simulink model "task1"  (R2024a)
settings: Solver=FixedStepAuto  StartTime=0.0  StopTime=10  FixedStep=0.001  RelTol=1e-3
settings Model: Creator=eva  LastModifiedBy=eva

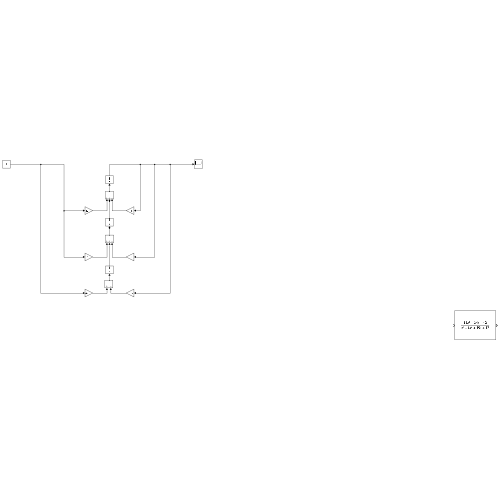
[thumbnail: Simulink's stored preview of the top-level diagram]
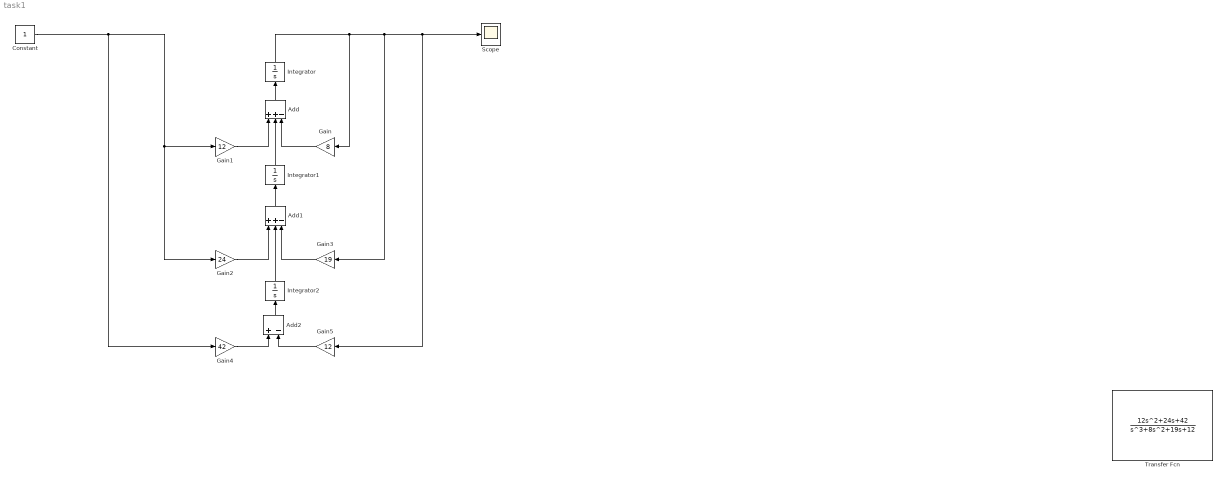
== system task1 ==
  Add : Sum  Inputs=++-
  Add1 : Sum  Inputs=++-
  Add2 : Sum  Inputs=+-
  Constant : Constant
  Gain : Gain  Gain=8
  Gain1 : Gain  Gain=12
  Gain2 : Gain  Gain=24
  Gain3 : Gain  Gain=19
  Gain4 : Gain  Gain=42
  Gain5 : Gain  Gain=12
  Integrator : Integrator
  Integrator1 : Integrator
  Integrator2 : Integrator
  Scope : Scope
  Transfer Fcn : TransferFcn  Numerator=[12 24 42]  Denominator=[1 8 19 12]
  wires:
  Integrator/1 -> Gain/1, Gain3/1, Gain5/1, Scope/1
  Constant/1 -> Gain4/1, Gain2/1, Gain1/1
  Gain1/1 -> Add/1
  Gain/1 -> Add/3
  Integrator1/1 -> Add/2
  Gain2/1 -> Add1/1
  Gain3/1 -> Add1/3
  Add/1 -> Integrator/1
  Integrator2/1 -> Add1/2
  Gain5/1 -> Add2/2
  Gain4/1 -> Add2/1
  Add1/1 -> Integrator1/1
  Add2/1 -> Integrator2/1
